simulink model "projekt1s"  (R2013a)
settings: Solver=ode45  StartTime=0.0  StopTime=10.0  RelTol=1e-3  AbsTol=1e-6
values from neighbouring files (symbols this model uses):
  cp = 1000    [projekt1.m]
  Cva = cp*rop*VaN    (= 3000)    [projekt1.m]
  Cvb = cp*rop*VbN    (= 135000)    [projekt1.m]
  dfwN = 0    [projekt1.m]
  dqgN = 0    [projekt1.m]
  dTzewN = 0    [projekt1.m]
  fwN = qgN*(TbN-TzewN)/(cp*rop*(TaN-TbN)*(TbN-TzewN)+cp*rop*(TaN-TbN)*(TaN-TzewN))    (= 0.729166666667)    [projekt1.m]
  Ka = (qgN-cp*rop*fwN*(TaN-TbN))/(TaN-TzewN)    (= 250)    [projekt1.m]
  Kb = (cp*rop*fwN*(TaN-TbN))/(TbN-TzewN)    (= 250)    [projekt1.m]
  qgN = 20000    [projekt1.m]
  rop = 1.2    [projekt1.m]
  TaN = 25    [projekt1.m]
  TbN = 15    [projekt1.m]
  ts = 1    [projekt1.m]
  TzewN = -20    [projekt1.m]
settings Model: Creator=LAB320-1552  LastModifiedBy=LAB320-1552
settings DebuggingCC: SolverPrmCheckMsg=none

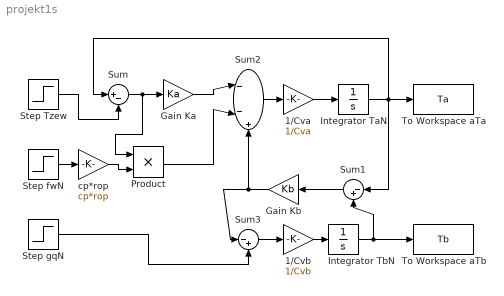
== system projekt1s ==
  1/Cva : Gain  Gain=1/Cva
  1/Cvb : Gain  Gain=1/Cvb
  Gain Ka : Gain  Gain=Ka
  Gain Kb : Gain  Gain=Kb
  Integrator TaN : Integrator  InitialCondition=TaN
  Integrator TbN : Integrator  InitialCondition=TbN
  Product : Product
  Step Tzew : Step  Time=ts  Before=TzewN  After=TzewN+dTzewN  SampleTime=0
  Step fwN : Step  Time=ts  Before=fwN  After=fwN+dfwN  SampleTime=0
  Step gqN : Step  Time=ts  Before=qgN  After=qgN+dqgN  SampleTime=0
  Sum : Sum  Inputs=|+-
  Sum1 : Sum  Inputs=|-+
  Sum2 : Sum  Inputs=|--+
  Sum3 : Sum  Inputs=|-+
  To Workspace aTa : ToWorkspace  VariableName=Ta  SampleTime=-1
  To Workspace aTb : ToWorkspace  VariableName=Tb  SampleTime=-1
  cp*rop : Gain  Gain=cp*rop
  wires:
  Step fwN/1 -> cp*rop/1
  cp*rop/1 -> Product/2
  Step Tzew/1 -> Sum/2
  Sum/1 -> Product/1, Gain Ka/1
  Gain Ka/1 -> Sum2/1
  Product/1 -> Sum2/2
  Step gqN/1 -> Sum3/2
  Gain Kb/1 -> Sum3/1, Sum2/3
  Sum3/1 -> 1/Cvb/1
  Sum2/1 -> 1/Cva/1
  1/Cvb/1 -> Integrator TbN/1
  1/Cva/1 -> Integrator TaN/1
  Integrator TbN/1 -> Sum1/2, To Workspace aTb/1
  Sum1/1 -> Gain Kb/1
  Integrator TaN/1 -> Sum1/1, Sum/1, To Workspace aTa/1
